simulink model "PhyMod_OpModeSelectNSync"  (R2016b)
settings: configuration reference "CodeGenConfigSet" (kept outside this file)
settings Model: Creator=Administrator  LastModifiedBy=Administrator
settings ConfigSetRef: SourceLocation=Base Workspace

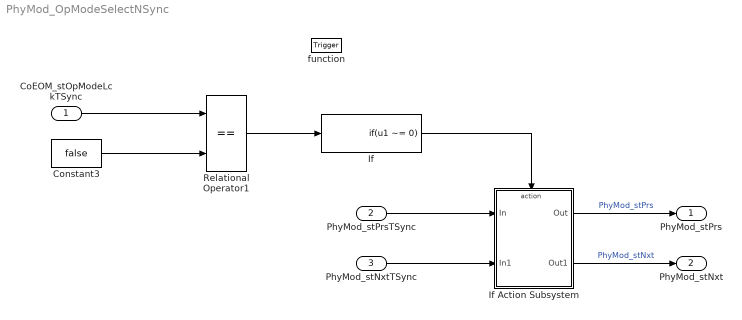
== system PhyMod_OpModeSelectNSync ==
  CoEOM_stOpModeLckTSync : Inport  Description=Status for synchronisation between time and engine speed synchronous tasks  OutMin=0  OutMax=1  OutDataTypeStr=boolean
  PhyMod_stPrsTSync : Inport  Description=Current operating mode for the torque structure (time synchronous)  Port=2  OutMin=0  OutMax=255  OutDataTypeStr=State_uint8
  PhyMod_stNxtTSync : Inport  Description=Next operating mode for the torque structure (time synchronous)  Port=3  OutMin=0  OutMax=255  OutDataTypeStr=State_uint8
  function : TriggerPort  TriggerType=function-call  VariantControl=Variant
  Constant3 : Constant  Value=false  OutDataTypeStr=boolean
  If : If  IfExpression=u1 ~= 0  ShowElse=off
  If Action Subsystem : Subsystem  TreatAsAtomicUnit=on
  Relational Operator1 : RelationalOperator  Operator===  OutDataTypeStr=boolean  RndMeth=Simplest  InputSameDT=on
  PhyMod_stPrs : Outport  Description=Current operating mode for the torque structure  OutMin=0  OutMax=255  OutDataTypeStr=State_uint8
  PhyMod_stNxt : Outport  Description=Next operating mode for the torque structure  Port=2  OutMin=0  OutMax=255  OutDataTypeStr=State_uint8
  wires:
  If Action Subsystem/2(Out1) -> PhyMod_stNxt/1  "PhyMod_stNxt"
  If/1 -> If Action Subsystem/Action
  PhyMod_stPrsTSync/1 -> If Action Subsystem/1(In)
  If Action Subsystem/1(Out) -> PhyMod_stPrs/1  "PhyMod_stPrs"
  PhyMod_stNxtTSync/1 -> If Action Subsystem/2(In1)
  Relational Operator1/1 -> If/1
  CoEOM_stOpModeLckTSync/1 -> Relational Operator1/1
  Constant3/1 -> Relational Operator1/2

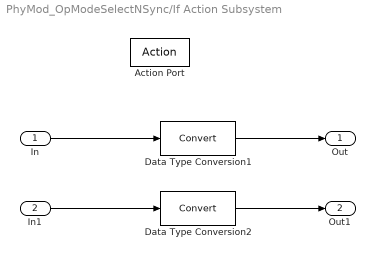
== system PhyMod_OpModeSelectNSync/If Action Subsystem ==
  In : Inport
  In1 : Inport  Port=2
  Action Port : ActionPort  ActionType=then
  Data Type Conversion1 : DataTypeConversion
  Data Type Conversion2 : DataTypeConversion
  Out : Outport
  Out1 : Outport  Port=2
  wires:
  Data Type Conversion2/1 -> Out1/1
  Data Type Conversion1/1 -> Out/1
  In1/1 -> Data Type Conversion2/1
  In/1 -> Data Type Conversion1/1
